simulink model "NavigationModel"  (R2025a)
settings: Solver=VariableStepAuto  StartTime=0.0  StopTime=10.0  FixedStep=0.01  RelTol=1e-3
libraries: simulink x12, slpidlib x2
settings Model: DataDictionary=Constants.sldd  Creator=levirogalla  LastModifiedBy=yaremadzulynsky

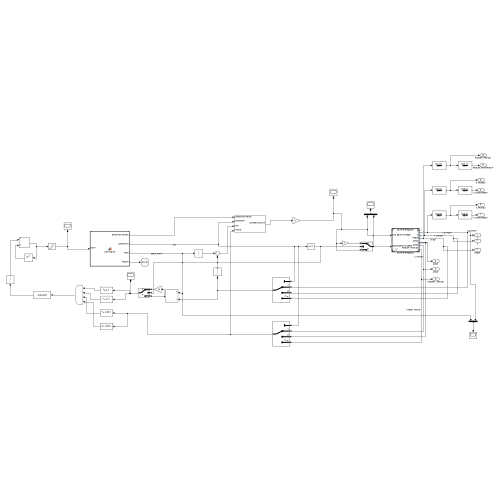
[thumbnail: Simulink's stored preview of the top-level diagram]
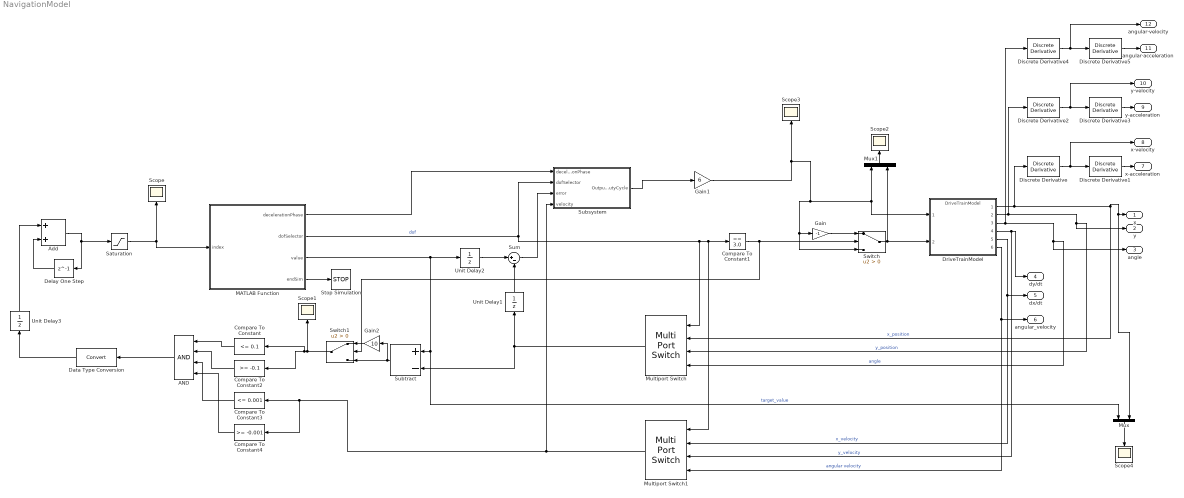
== system NavigationModel ==
  AND : Logic  Inputs=4  IconShape=distinctive  AllPortsSameDT=off  OutDataTypeStr=boolean
  Add : Sum
  Compare To Constant : simulink/Logic and Bit Operations/Compare To Constant  relop=<=  const=0.1  OutDataTypeStr=boolean
  Compare To Constant1 : simulink/Logic and Bit Operations/Compare To Constant  relop===  const=3.0  OutDataTypeStr=boolean
  Compare To Constant2 : simulink/Logic and Bit Operations/Compare To Constant  relop=>=  const=-0.1  OutDataTypeStr=boolean
  Compare To Constant3 : simulink/Logic and Bit Operations/Compare To Constant  relop=<=  const=0.001  OutDataTypeStr=boolean
  Compare To Constant4 : simulink/Logic and Bit Operations/Compare To Constant  relop=>=  const=-0.001  OutDataTypeStr=boolean
  Data Type Conversion : DataTypeConversion  SaturateOnIntegerOverflow=off  RndMeth=Floor
  Delay One Step : Delay  DelayLength=1
  Discrete Derivative{,1..5} (6 alike) : simulink/Discrete/Discrete Derivative  gainval=1.0  ICPrevScaledInput=0.0  OutMin=[]  OutMax=[]  OutDataType=fixdt(1, 16)  OutScaling=2^-10  DoSatur=off
  DriveTrainModel : ModelReference  ModelNameDialog=DriveTrainModel.slx  SimulationMode=Normal  ModelReferenceVersion=1.10
  Gain : Gain  Gain=-1
  Gain1 : Gain  Gain=6
  Gain2 : Gain  Gain=10
  MATLAB Function : MATLAB Function  TreatAsAtomicUnit=on
  Multiport Switch : MultiPortSwitch  SaturateOnIntegerOverflow=off  InputSameDT=off
  Multiport Switch1 : MultiPortSwitch  SaturateOnIntegerOverflow=off  InputSameDT=off
  Mux : Mux  Inputs=2
  Mux1 : Mux  Inputs=2
  Saturation : Saturate  UpperLimit=5  LowerLimit=0  LinearizeAsGain=off
  Scope{,1..4} (5 alike) : Scope
      Scope settings: ActiveDisplayYMinimum=-0.125  ActiveDisplayYMaximum=1.125
      Scope1 settings: ActiveDisplayYMinimum=-22.01338  ActiveDisplayYMaximum=19.1126  DataLoggingVariableName=ScopeData5
      Scope2 settings: ActiveDisplayYMinimum=-7.754803792300577  ActiveDisplayYMaximum=1.1949781991445083  DataLoggingVariableName=ScopeData6
      Scope3 settings: ActiveDisplayYMinimum=-1.5  ActiveDisplayYMaximum=13.5  DataLoggingVariableName=ScopeData7
      Scope4 settings: ActiveDisplayYMinimum=-3.7664036777078795  ActiveDisplayYMaximum=18.189669831421952
  Stop Simulation : Stop
  Subsystem : Subsystem
  Subtract : Sum  Inputs=+-
  Sum : Sum  Inputs=|+-
  Switch : Switch  Criteria=u2 > Threshold  SaturateOnIntegerOverflow=off  InputSameDT=off
  Switch1 : Switch  Criteria=u2 > Threshold  SaturateOnIntegerOverflow=off  InputSameDT=off
  Unit Delay1 : UnitDelay  SampleTime=-1  HasFrameUpgradeWarning=on
  Unit Delay2 : UnitDelay  SampleTime=-1  HasFrameUpgradeWarning=on
  Unit Delay3 : UnitDelay  SampleTime=-1  HasFrameUpgradeWarning=on
  x : Outport
  y : Outport  Port=2
  angle : Outport  Port=3
  dy/dt : Outport  Port=4
  dx/dt : Outport  Port=5
  angular_velocity : Outport  Port=6
  x-acceleration : Outport  Port=7
  x-velocity : Outport  Port=8
  y-acceleration : Outport  Port=9
  y-velocity : Outport  Port=10
  angular-acceleration : Outport  Port=11
  angular-velocity : Outport  Port=12
  wires:
  Multiport Switch/1 -> Subtract/2, Unit Delay1/1
  Compare To Constant/1 -> AND/1
  Add/1 -> Delay One Step/1, Saturation/1
  Delay One Step/1 -> Add/2
  Compare To Constant2/1 -> AND/2
  MATLAB Function/2(dofSelector) -> Subsystem/2(dofSelector), Multiport Switch/1, Multiport Switch1/1, Compare To Constant1/1  "dof"
  Switch/1 -> DriveTrainModel/2, Mux1/2
  Gain/1 -> Switch/1
  MATLAB Function/3(value) -> Subtract/1, Mux/1, Unit Delay2/1  "target_value"
  Saturation/1 -> MATLAB Function/1(index), Scope/1
  DriveTrainModel/3 -> Discrete Derivative4/1, angle/1, Multiport Switch/4  "angle"
  Mux1/1 -> Scope2/1
  DriveTrainModel/1 -> Discrete Derivative/1, Mux/2, x/1, Multiport Switch/2  "x_position"
  AND/1 -> Data Type Conversion/1
  DriveTrainModel/2 -> Discrete Derivative2/1, y/1, Multiport Switch/3  "y_position"
  Gain1/1 -> Mux1/1, DriveTrainModel/1, Switch/3, Gain/1, Scope3/1
  Data Type Conversion/1 -> Unit Delay3/1
  MATLAB Function/4(endSim) -> Stop Simulation/1
  Compare To Constant1/1 -> Switch1/2, Switch/2
  Unit Delay3/1 -> Add/1
  Sum/1 -> Subsystem/3(error)
  Subsystem/1(OutputDutyCycle) -> Gain1/1
  MATLAB Function/1(decelerationPhase) -> Subsystem/1(decelerationPhase)
  Mux/1 -> Scope4/1
  DriveTrainModel/4 -> Multiport Switch1/3, dy/dt/1  "y_velocity"
  DriveTrainModel/5 -> Multiport Switch1/2, dx/dt/1  "x_velocity"
  Unit Delay1/1 -> Sum/2
  DriveTrainModel/6 -> angular_velocity/1, Multiport Switch1/4  "angular velocity"
  Multiport Switch1/1 -> Subsystem/4(velocity), Compare To Constant4/1, Compare To Constant3/1
  Compare To Constant3/1 -> AND/3
  Compare To Constant4/1 -> AND/4
  Unit Delay2/1 -> Sum/1
  Subtract/1 -> Gain2/1, Switch1/3
  Switch1/1 -> Scope1/1, Compare To Constant/1, Compare To Constant2/1
  Gain2/1 -> Switch1/1
  Discrete Derivative/1 -> x-velocity/1, Discrete Derivative1/1
  Discrete Derivative1/1 -> x-acceleration/1
  Discrete Derivative3/1 -> y-acceleration/1
  Discrete Derivative2/1 -> Discrete Derivative3/1, y-velocity/1
  Discrete Derivative4/1 -> angular-velocity/1, Discrete Derivative5/1
  Discrete Derivative5/1 -> angular-acceleration/1

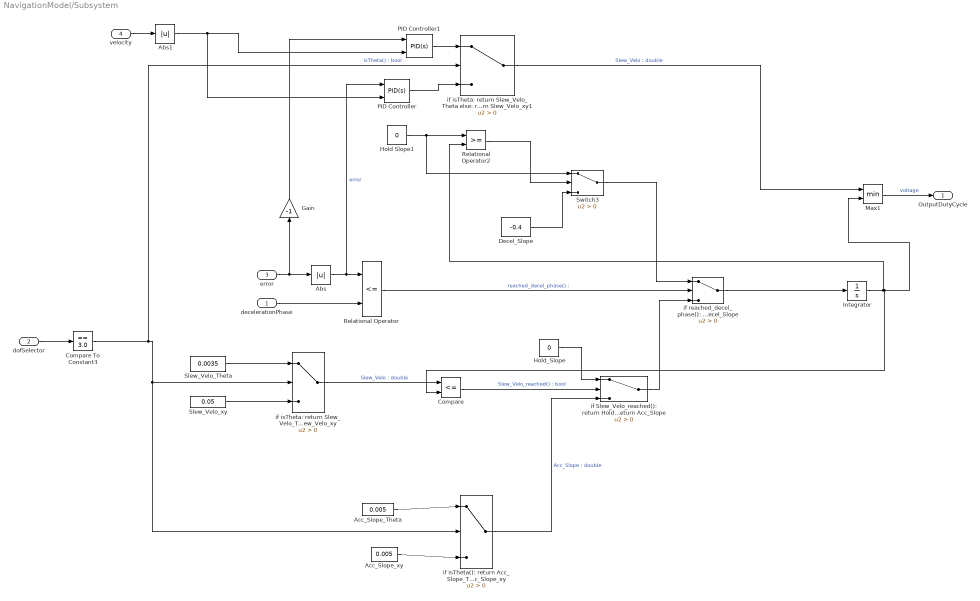
== system NavigationModel/Subsystem ==
  decelerationPhase : Inport
  dofSelector : Inport  Port=2
  error : Inport  Port=3
  velocity : Inport  Port=4
  Abs : Abs  SaturateOnIntegerOverflow=off
  Abs1 : Abs  SaturateOnIntegerOverflow=off
  Acc_Slope_Theta : Constant  Value=0.005
  Acc_Slope_xy : Constant  Value=0.005
  "Compare " : RelationalOperator  Operator=<=  OutDataTypeStr=boolean  RndMeth=Simplest  InputSameDT=off
  Compare To Constant3 : simulink/Logic and Bit Operations/Compare To Constant  relop===  const=3.0  OutDataTypeStr=boolean
  Decel_Slope : Constant  Value=-0.4
  Gain : Gain  Gain=-1
  "Hold Slope1 " : Constant  Value=0
  Hold_Slope : Constant  Value=0
  Integrator : Integrator
  Max1 : MinMax  Inputs=2
  PID Controller : slpidlib/PID Controller  Controller=PID  Form=Parallel  TimeDomain=Continuous-time  UseExternalTs=off  SampleTime=-1  IntegratorMethod=Forward Euler  FilterMethod=Forward Euler  ControllerParametersSource=internal  P=2  I=0  UseKiTs=off  D=8  UseExternalDerivativeSource=on  N=100  UseFilter=on  TunerSelectOption=Transfer Function Based (PID Tuner App)  InitialConditionSource=internal  InitialConditionForIntegrator=0  InitialConditionForFilter=0  DifferentiatorICPrevScaledInput=0  ExternalReset=none  TrackingMode=off  Kt=1  LimitOutput=off  SatLimitsSource=internal  UpperSaturationLimit=inf  LowerSaturationLimit=-inf  LinearizeAsGain=on  AntiWindupMode=none  Kb=1  LimitIntegrator=off  UpperIntegratorSaturationLimit=inf  LowerIntegratorSaturationLimit=-inf  POutMin=[]  POutMax=[]  IOutMin=[]  IOutMax=[]  DOutMin=[]  DOutMax=[]  NOutMin=[]  NOutMax=[]  SumOutMin=[]  SumOutMax=[]  SaturationOutMin=[]  SaturationOutMax=[]  PParamMin=[]  PParamMax=[]  IParamMin=[]  IParamMax=[]  DParamMin=[]  DParamMax=[]  NParamMin=[]  NParamMax=[]  KbParamMin=[]  KbParamMax=[]  KtParamMin=[]  KtParamMax=[]  KbOutMin=[]  KbOutMax=[]  KtOutMin=[]  KtOutMax=[]  IntegratorOutMin=[]  IntegratorOutMax=[]  FilterOutMin=[]  FilterOutMax=[]  SumI1OutMin=[]  SumI1OutMax=[]  SumI2OutMin=[]  SumI2OutMax=[]  SumI3OutMin=[]  SumI3OutMax=[]  SumI4OutMin=[]  SumI4OutMax=[]  SumDOutMin=[]  SumDOutMax=[]  DifferentiatorOutMin=[]  DifferentiatorOutMax=[]  FilterDiffOutCoefMin=[]  FilterDiffOutCoefMax=[]  ReciprocalOutMin=[]  ReciprocalOutMax=[]  SumDenOutMin=[]  SumDenOutMax=[]  SumNumOutMin=[]  SumNumOutMax=[]  DivideOutMin=[]  DivideOutMax=[]  UdiffTsProdOutMin=[]  UdiffTsProdOutMax=[]  NTsProdOutMin=[]  NTsProdOutMax=[]  UintegralTsProdOutMin=[]  UintegralTsProdOutMax=[]  UngainTsProdOutMin=[]  UngainTsProdOutMax=[]  ClampingZeroOutDataTypeStr=Inherit: Inherit via back propagation  ClampingZeroOutMin=[]  ClampingZeroOutMax=[]  FilterDenConstantOutDataTypeStr=Inherit: Inherit via back propagation  FilterDenConstantOutMin=[]  FilterDenConstantOutMax=[]  PCopyOutDataTypeStr=Inherit: Inherit via back propagation  PCopyOutMin=[]  PCopyOutMax=[]  NCopyOutDataTypeStr=Inherit: Inherit via back propagation  NCopyOutMin=[]  NCopyOutMax=[]  IntegratorContinuousStateAttributes=''  IntegratorStateMustResolveToSignalObject=off  IntegratorRTWStateStorageClass=Auto  FilterContinuousStateAttributes=''  FilterStateMustResolveToSignalObject=off  FilterRTWStateStorageClass=Auto  ParallelPVariant=InternalParameters  IdealPVariant=Disabled  IVariant=InternalParameters  DVariant=InternalParameters  IntegratorVariant=Continuous  SatVariant=Disabled  AWVariant=Passthrough  PCopyVariant=Disabled  TRVariant=Disabled  FdbkBlocksVariant=Forward  IdealPFdbkVariant=Disabled  SatFdbkVariant=Disabled  DerivativeFilterVariant=ContFilterOnly  NVariant=InternalParameters  NCopyVariant=Disabled  FilterICVariant=InternalICsFilter  IntegratorICVariant=InternalICs  ExternalResetVariant=Disabled  TRSumVariant=Passthrough  SumFdbkVariant=Disabled  SumVariant=Sum_PID  TsampFilterVariant=InternalTs  TsampNgainVariant=Passthrough  TsampIntegralVariant=Disabled_SignalSpec  ExternalSaturationOutDataTypeStr=Inherit: Same as second input  DerivativeSourceVariant=ExternalYdot  PreIntVariant=InternalPreInt
  PID Controller1 : slpidlib/PID Controller  Controller=PID  Form=Parallel  TimeDomain=Continuous-time  UseExternalTs=off  SampleTime=-1  IntegratorMethod=Forward Euler  FilterMethod=Forward Euler  ControllerParametersSource=internal  P=0.5  I=0  UseKiTs=off  D=4  UseExternalDerivativeSource=on  N=100  UseFilter=on  TunerSelectOption=Transfer Function Based (PID Tuner App)  InitialConditionSource=internal  InitialConditionForIntegrator=0  InitialConditionForFilter=0  DifferentiatorICPrevScaledInput=0  ExternalReset=none  TrackingMode=off  Kt=1  LimitOutput=off  SatLimitsSource=internal  UpperSaturationLimit=inf  LowerSaturationLimit=-inf  LinearizeAsGain=on  AntiWindupMode=none  Kb=1  LimitIntegrator=off  UpperIntegratorSaturationLimit=inf  LowerIntegratorSaturationLimit=-inf  POutMin=[]  POutMax=[]  IOutMin=[]  IOutMax=[]  DOutMin=[]  DOutMax=[]  NOutMin=[]  NOutMax=[]  SumOutMin=[]  SumOutMax=[]  SaturationOutMin=[]  SaturationOutMax=[]  PParamMin=[]  PParamMax=[]  IParamMin=[]  IParamMax=[]  DParamMin=[]  DParamMax=[]  NParamMin=[]  NParamMax=[]  KbParamMin=[]  KbParamMax=[]  KtParamMin=[]  KtParamMax=[]  KbOutMin=[]  KbOutMax=[]  KtOutMin=[]  KtOutMax=[]  IntegratorOutMin=[]  IntegratorOutMax=[]  FilterOutMin=[]  FilterOutMax=[]  SumI1OutMin=[]  SumI1OutMax=[]  SumI2OutMin=[]  SumI2OutMax=[]  SumI3OutMin=[]  SumI3OutMax=[]  SumI4OutMin=[]  SumI4OutMax=[]  SumDOutMin=[]  SumDOutMax=[]  DifferentiatorOutMin=[]  DifferentiatorOutMax=[]  FilterDiffOutCoefMin=[]  FilterDiffOutCoefMax=[]  ReciprocalOutMin=[]  ReciprocalOutMax=[]  SumDenOutMin=[]  SumDenOutMax=[]  SumNumOutMin=[]  SumNumOutMax=[]  DivideOutMin=[]  DivideOutMax=[]  UdiffTsProdOutMin=[]  UdiffTsProdOutMax=[]  NTsProdOutMin=[]  NTsProdOutMax=[]  UintegralTsProdOutMin=[]  UintegralTsProdOutMax=[]  UngainTsProdOutMin=[]  UngainTsProdOutMax=[]  ClampingZeroOutDataTypeStr=Inherit: Inherit via back propagation  ClampingZeroOutMin=[]  ClampingZeroOutMax=[]  FilterDenConstantOutDataTypeStr=Inherit: Inherit via back propagation  FilterDenConstantOutMin=[]  FilterDenConstantOutMax=[]  PCopyOutDataTypeStr=Inherit: Inherit via back propagation  PCopyOutMin=[]  PCopyOutMax=[]  NCopyOutDataTypeStr=Inherit: Inherit via back propagation  NCopyOutMin=[]  NCopyOutMax=[]  IntegratorContinuousStateAttributes=''  IntegratorStateMustResolveToSignalObject=off  IntegratorRTWStateStorageClass=Auto  FilterContinuousStateAttributes=''  FilterStateMustResolveToSignalObject=off  FilterRTWStateStorageClass=Auto  ParallelPVariant=InternalParameters  IdealPVariant=Disabled  IVariant=InternalParameters  DVariant=InternalParameters  IntegratorVariant=Continuous  SatVariant=Disabled  AWVariant=Passthrough  PCopyVariant=Disabled  TRVariant=Disabled  FdbkBlocksVariant=Forward  IdealPFdbkVariant=Disabled  SatFdbkVariant=Disabled  DerivativeFilterVariant=ContFilterOnly  NVariant=InternalParameters  NCopyVariant=Disabled  FilterICVariant=InternalICsFilter  IntegratorICVariant=InternalICs  ExternalResetVariant=Disabled  TRSumVariant=Passthrough  SumFdbkVariant=Disabled  SumVariant=Sum_PID  TsampFilterVariant=InternalTs  TsampNgainVariant=Passthrough  TsampIntegralVariant=Disabled_SignalSpec  ExternalSaturationOutDataTypeStr=Inherit: Same as second input  DerivativeSourceVariant=ExternalYdot  PreIntVariant=InternalPreInt
  Relational Operator : RelationalOperator  Operator=<=  OutDataTypeStr=boolean  RndMeth=Simplest  InputSameDT=off
  Relational Operator2 : RelationalOperator  OutDataTypeStr=boolean  RndMeth=Simplest  InputSameDT=off
  Slew_Velo_Theta : Constant  Value=0.0035
  Slew_Velo_xy : Constant  Value=0.05
  Switch3 : Switch  Criteria=u2 > Threshold  SaturateOnIntegerOverflow=off  InputSameDT=off
  if Slew_Velo_reached(): return Hold_Slope else: return Acc_Slope : Switch  Criteria=u2 > Threshold  SaturateOnIntegerOverflow=off  InputSameDT=off
  if isTheta(): return Acc_Slope_Theta else: return Acc_Slope_xy : Switch  Criteria=u2 > Threshold  SaturateOnIntegerOverflow=off  InputSameDT=off
  if isTheta: return Slew_Velo_Theta else: return Slew_Velo_xy : Switch  Criteria=u2 > Threshold  SaturateOnIntegerOverflow=off  InputSameDT=off
  if isTheta: return Slew_Velo_Theta else: return Slew_Velo_xy1 : Switch  Criteria=u2 > Threshold  SaturateOnIntegerOverflow=off  InputSameDT=off
  "if reached_decel_phase(): return Decel_Slope " : Switch  Criteria=u2 > Threshold  SaturateOnIntegerOverflow=off  InputSameDT=off
  OutputDutyCycle : Outport
  wires:
  "Hold Slope1 "/1 -> Switch3/1, Relational Operator2/1
  Switch3/1 -> "if reached_decel_phase(): return Decel_Slope "/1
  if isTheta: return Slew_Velo_Theta else: return Slew_Velo_xy/1 -> "Compare "/1  "Slew_Velo : double"
  Compare To Constant3/1 -> if isTheta: return Slew_Velo_Theta else: return Slew_Velo_xy1/2, if isTheta(): return Acc_Slope_Theta else: return Acc_Slope_xy/2, if isTheta: return Slew_Velo_Theta else: return Slew_Velo_xy/2  "isTheta() : bool"
  Slew_Velo_Theta/1 -> if isTheta: return Slew_Velo_Theta else: return Slew_Velo_xy/1
  if isTheta(): return Acc_Slope_Theta else: return Acc_Slope_xy/1 -> if Slew_Velo_reached(): return Hold_Slope else: return Acc_Slope/3  "Acc_Slope : double"
  Slew_Velo_xy/1 -> if isTheta: return Slew_Velo_Theta else: return Slew_Velo_xy/3
  Acc_Slope_Theta/1 -> if isTheta(): return Acc_Slope_Theta else: return Acc_Slope_xy/1
  Relational Operator2/1 -> Switch3/2
  "Compare "/1 -> if Slew_Velo_reached(): return Hold_Slope else: return Acc_Slope/2  "Slew_Velo_reached() : bool"
  Acc_Slope_xy/1 -> if isTheta(): return Acc_Slope_Theta else: return Acc_Slope_xy/3
  Abs/1 -> PID Controller/1, Relational Operator/1  "error"
  Decel_Slope/1 -> Switch3/3
  Relational Operator/1 -> "if reached_decel_phase(): return Decel_Slope "/2  "reached_decel_phase() :"
  if Slew_Velo_reached(): return Hold_Slope else: return Acc_Slope/1 -> "if reached_decel_phase(): return Decel_Slope "/3
  "if reached_decel_phase(): return Decel_Slope "/1 -> Integrator/1
  Hold_Slope/1 -> if Slew_Velo_reached(): return Hold_Slope else: return Acc_Slope/1
  decelerationPhase/1 -> Relational Operator/2
  error/1 -> Abs/1, Gain/1
  dofSelector/1 -> Compare To Constant3/1
  Max1/1 -> OutputDutyCycle/1  "voltage"
  PID Controller/1 -> if isTheta: return Slew_Velo_Theta else: return Slew_Velo_xy1/3
  if isTheta: return Slew_Velo_Theta else: return Slew_Velo_xy1/1 -> Max1/1  "Slew_Velo : double"
  Integrator/1 -> Max1/2, "Compare "/2, Relational Operator2/2
  PID Controller1/1 -> if isTheta: return Slew_Velo_Theta else: return Slew_Velo_xy1/1
  velocity/1 -> Abs1/1
  Abs1/1 -> PID Controller/2, PID Controller1/2
  Gain/1 -> PID Controller1/1

== matlab function NavigationModel/MATLAB Function ==
  data: decelerationPhase output; dofSelector output; value output; index input; endSim output
function [decelerationPhase, dofSelector, value, endSim] = pathSignal(index)
% Returns path values and a signal to stop simulation when out of bounds

% Define the path matrix
pathMatrix = [
    15, 1, 3;
    -pi/2, 3, 1;
    -10, 2, 3.8;
    -pi, 3, 1;
    8, 1, 3
              ];

% Get the size of the path
N = size(pathMatrix, 1);

% Initialize outputs
value = 0;
dofSelector = 1;
decelerationPhase = 0;
endSim = false;

% Check if index is within bounds
if index + 1 <= N
    value = pathMatrix(index + 1, 1);
    dofSelector = pathMatrix(index + 1, 2);
    decelerationPhase = pathMatrix(index + 1, 3);
else
    endSim = true;  % signal to stop the simulation
end
